simulink model "Lab1"  (R2021a)
settings: Solver=VariableStepAuto  StartTime=0.0  StopTime=10.0  RelTol=1e-3
settings Model: Creator=hp  LastModifiedBy=hp

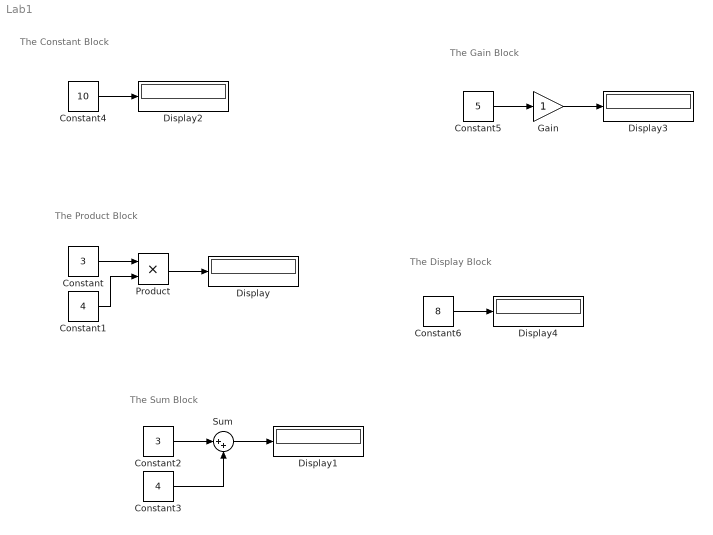
== system Lab1 ==
  note: The Constant Block
  note: The Sum Block
  note: The Product Block
  note: The Gain Block
  note: The Display Block
  Constant : Constant  Value=3
  Constant1 : Constant  Value=4
  Constant2 : Constant  Value=3
  Constant3 : Constant  Value=4
  Constant4 : Constant  Value=10
  Constant5 : Constant  Value=5
  Constant6 : Constant  Value=8
  Display{,1..4} (5 alike) : Display
  Gain : Gain
  Product : Product
  Sum : Sum  Inputs=|++
  wires:
  Constant4/1 -> Display2/1
  Sum/1 -> Display1/1
  Constant/1 -> Product/1
  Constant3/1 -> Sum/2
  Constant1/1 -> Product/2
  Product/1 -> Display/1
  Constant2/1 -> Sum/1
  Constant5/1 -> Gain/1
  Gain/1 -> Display3/1
  Constant6/1 -> Display4/1
